simulink model "simulation code"  (R2023a)
settings: Solver=VariableStepAuto  StartTime=0.0  StopTime=1  MaxStep=1e-6  RelTol=1e-3
InitFcn:
  | Ts=1/1550;
undefined symbols (not defined in the file): powergui, sps_lib
libraries: spsIGBTDiodeLib x6, spsVoltageMeasurementLib x6, spsabctoAlphaBetaZeroLib x2, spsDCVoltageSourceLib x1, spsGroundLib x1, simulink x1, simulink_extras x1, spspowerguiLib x1, spsThreePhaseSeriesRLCBranchLib x1, spsThreePhaseVIMeasurementLib x1
settings DataIOCC: ReturnWorkspaceOutputs=off

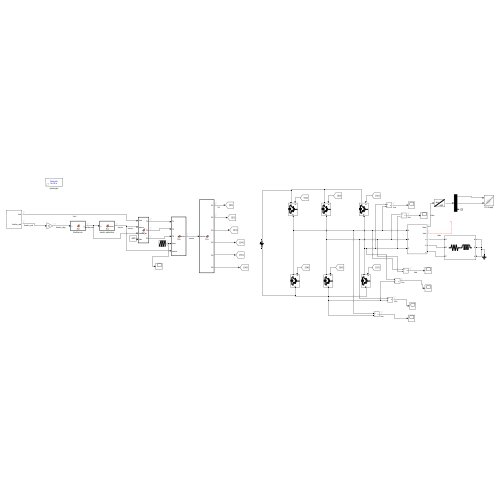
[thumbnail: Simulink's stored preview of the top-level diagram]
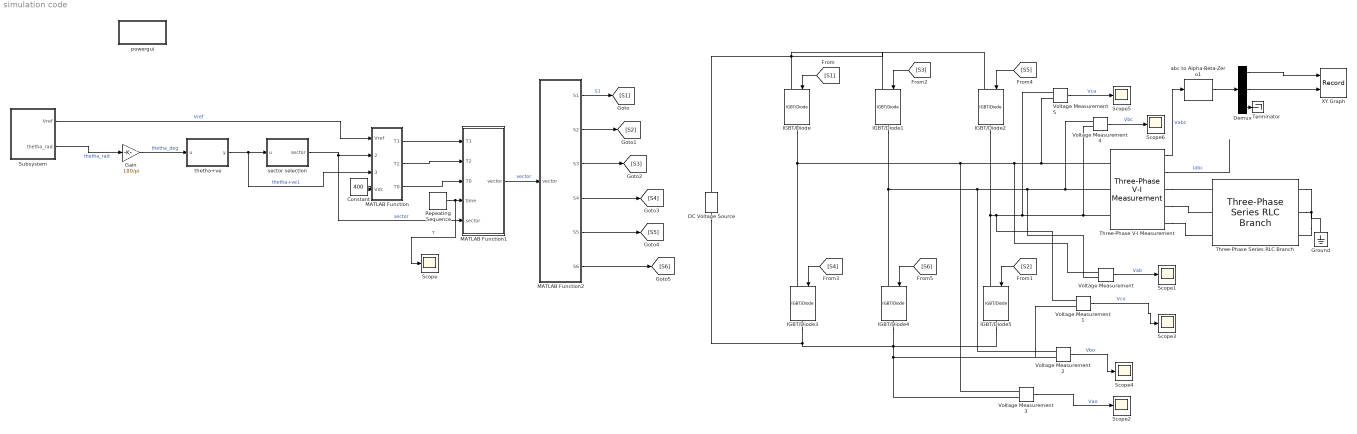
== system simulation code ==
  Constant : Constant  Value=400
  DC Voltage Source : spsDCVoltageSourceLib/DC Voltage Source  Amplitude=400  Measurements=None
  Demux : Demux  Outputs=3
  Gain : Gain  Gain=180/pi
  Ground : spsGroundLib/Ground  LConnTagsString=a
  IGBT/Diode{,1..5} (6 alike) : spsIGBTDiodeLib/IGBT//Diode  Ron=1e-3  Rs=1e5  Cs=inf  Measurements=off
  MATLAB Function : MATLAB Function  TreatAsAtomicUnit=on
  MATLAB Function1 : MATLAB Function  TreatAsAtomicUnit=on
  MATLAB Function2 : MATLAB Function  TreatAsAtomicUnit=on
  Repeating Sequence : simulink/Sources/Repeating Sequence  rep_seq_t=[0 1]*Ts  rep_seq_y=[0 Ts]
  Scope{,1..6} (7 alike) : Scope
  Subsystem : Subsystem
  Terminator : Terminator
  Three-Phase Series RLC Branch : spsThreePhaseSeriesRLCBranchLib/Three-Phase Series RLC Branch  LConnTagsString=A|B|C  RConnTagsString=A|B|C  BranchType=RL  Resistance=1  Inductance=1e-2  Capacitance=0  Measurements=None
  Three-Phase V-I Measurement : spsThreePhaseVIMeasurementLib/Three-Phase V-I Measurement  VoltageMeasurement=phase-to-ground  SetLabelV=off  LabelV=Vabc  Vpu=off  VpuLL=off  CurrentMeasurement=yes  SetLabelI=off  LabelI=Iabc  Ipu=off  Pbase=100e6  Vbase=500e3  OutputType=Complex  PhasorSimulation=off  PSBequivalent=0
  Voltage Measurement{,1..5} (6 alike) : spsVoltageMeasurementLib/Voltage Measurement  PhasorSimulation=off  OutputType=Complex  PSBequivalent=0
  XY Graph : Record  FileSettingsInternal="{\"entries\":[{\"content\":{\"excelSettings\":{\"content\":{},\"type\":\"Streamout.ExcelSettings\"}},\"type\":\"Streamout.FileSettingStorage\",\"uuid\":\"\"}],\"packageUris\":[\"http:\\/\\/schema.mathworks.com\\/mf0\\/streamout_blocks\\/R2020a\"],\"version\":\"1.0\"}"  Layout=[1 1]  SignalsInternal="{\"entries\":[{\"content\":{\"signals\":[{\"content\":{\"blockPath\":[],\"dimensions\":[1],\"domain\":\"\",\"lineColor\":\"#77ac30\",\"plots\":[1],\"port\":1,\"signalID\":12102,\"signalName\":\"Demux:1\"},\"type\":\"RecordBlkView.Signal\",\"uuid\":\"\"},{\"content\":{\"blockPath\":[],\"dimensions\":[1],\"domain\":\"\",\"lineColor\":\"#139fff\",\"plots\":[1],\"port\":2,\"signalID\":12105,\"signalName\":\"Demux:2\"},\"type\":\"RecordBlkView.Signal\",\"uuid\":\"\"}]},\"type\":\"RecordBlkView.InputSignals\",\"uuid\":\"\"}],\"packageUris\":[\"http:\\/\\/schema.mathworks.com\\/mf0\\/streamout_blocks\\/R2020a\"],\"version\":\"1.0\"}"  VisualizationBindings="{\"xyplotplugin\":{\"info\":[{\"series\":[{\"bindingParametersList\":[{\"parameter\":\"X-Axis\",\"signalID\":12102,\"signalName\":\"Demux:1\"},{\"parameter\":\"Y-Axis\",\"signalID\":12105,\"signalName\":\"Demux:2\"}],\"seriesID\":46144}],\"subplotID\":1}]}}"  CompatibilityTag=XY  st=-1
  abc to Alpha-Beta-Zero1 : spsabctoAlphaBetaZeroLib/abc to Alpha-Beta-Zero
  powergui : Subsystem  Priority=1  AncestorBlock=sps_lib/powergui  DialogController=POWERSYS.PowerSysDialog  InitFcn=powergui( 'InitFcn_Callback' , gcb , 0 , [ ] );  mask(PSB option menu block){SimulationMode=Discrete, SampleTime=50e-6, frequency=60, Iterations=50, frequencyindice=0, Pbase=100e6, ErrMax=1e-4, UnitsV=kV, UnitsW=MW, buscounter=0, FunctionMessages=off, echomessages=off, EnableUseOfTLC=off, CurrentSourceSwitches=off, DisableSnubberDevices=off, DisableRonSwitches=off, DisableVfSwitches=off, DisplayEquations=off, AutomaticDiscreteSolvers=off, SolverType=Tustin/Backward Euler (TBE), Interpol=off, ExternalGateDelay=off, methode=off, Ts=100, x0status=blocks, SPID=on, SwTol=0, HookPort=off, NonlinearTolerance=1e-4, nMaxIteration=100, ContinueOnMaxIteration=off, RestoreLinks=warning, ResistiveCurrentMeasurement=off, Frange=[0:2:500], Ylog=off, Xlog=on, ShowGrid=off, save=off, variable=ZData, structure=0, ZoomFFT=off, StartTime=0.0, cycles=1, DisplayStyle=1, fundamental=60, FreqAxis=off, MaxFrequency=1000, frequencyindicesteady=1, RmsSteady=1, display=off}
      mask prompts: SimulationMode "Simulation type:"; SampleTime "Sample time (s):"; frequency "Frequency (Hz):"; Iterations "Max iterations"; frequencyindice "Frequency (Hz)"; Pbase "Base power (VA)"; ErrMax "PQ tolerance (pu)"; UnitsV "Voltage units"; UnitsW "Power units"; buscounter "Load flow bus counter"; FunctionMessages "Disable Specialized Power Systems warnings"; echomessages "Display Specialized Power Systems compilation messages"; EnableUseOfTLC "Use TLC file when in Accelerator Simulation Mode and for code generation"; CurrentSourceSwitches "Disable ideal switching"; DisableSnubberDevices "Disable snubbers in switching devices"; DisableRonSwitches "Disable Ron resistances in switching devices"; DisableVfSwitches "Disable forward voltages in switching devices"; DisplayEquations "Display circuit differential equations"; AutomaticDiscreteSolvers "Automatically handle Discrete solver and Advanced tab solver settings of blocks"; SolverType "Discrete solver"; Interpol "Interpolate switching events"; ExternalGateDelay "Use time-stamped gate signals"; methode "Store switching topologies"; Ts "Buffer size (MBytes):"; x0status "Start simulation with initial electrical states from:"; SPID "Use ideal switching devices"; SwTol "Switch tolerance"; HookPort "Allow multiple powergui blocks"; NonlinearTolerance "Solver tolerance"; nMaxIteration "Maximum number of iterations"; ContinueOnMaxIteration "Continue Simulation if maximum number of iterations is reached"; RestoreLinks "Restore disabled links of Simscape Power Systems ST blocks:"; ResistiveCurrentMeasurement "Use non ideal current measurement blocks (1e-4Ohm internal resistance)"; Frange "Frequency Range"; Ylog "Log impedance"; Xlog "log Frequency"; ShowGrid "grid"; save "Save Data To Workspace"; variable "Variable Name"; structure "Structure Name (PSBFFTSCOPE)"; ZoomFFT "ZoomFFT (PSBFFTSCOPE)"; StartTime "Start Time (PSBFFTSCOPE)"; cycles "Cycles (PSBFFTSCOPE)"; DisplayStyle "Display style (PSBFFTSCOPE)"; fundamental "Fundamental (PSBFFTSCOPE)"; FreqAxis "Frequency Axis (PSBFFTSCOPE)"; MaxFrequency "Max Frequency (PSBFFTSCOPE)"; frequencyindicesteady "Frequency indice (STEADYSTATE)"; RmsSteady "RMS display (STEADYSTATE)"; display "Display Results"
      mask help: Set simulation type, simulation parameters, and preferences.
      mask init:
      | dispMessage = '';
      | dispMessage = powergui('MaskInitialization',gcb,SimulationMode,SampleTime);
      settings: LibrarySourceBlock=sps_lib/powergui  PreSaveFcn=powergui( 'PreSaveFcn_Callback' , gcb , [ ] , [ ] );  OpenFcn=sps_rtmsupport('OpenFcn',gcbh)
      mask Help: helpview(psbhelp)
      mask TypeOptions SimulationMode: Continuous | Discrete | Phasor | Discrete phasor
      mask Callback SimulationMode: powergui('SimulationType',[],[],gcb);
      mask TypeOptions UnitsV: V | kV
      mask TypeOptions UnitsW: W | kW | MW
      mask Callback CurrentSourceSwitches: powergui('SimulationType',[],[],gcb);
      mask Callback AutomaticDiscreteSolvers: powergui('SimulationType',[],[],gcb);
      mask TypeOptions SolverType: Tustin/Backward Euler (TBE) | Tustin | Backward Euler
      mask Callback SolverType: powergui('SimulationType',[],[],gcb);
      mask Callback Interpol: powergui('SimulationType',[],[],gcb);
      mask Callback ExternalGateDelay: powergui('SimulationType',[],[],gcb);
      mask Callback methode: powergui('SimulationType',[],[],gcb);
      mask TypeOptions x0status: blocks | steady | zero
      mask TypeOptions RestoreLinks: yes | warning | no
      mask Callback display: sps_rtmsupport('parametereditingmodes',gcbh) % Will be executed last in parameter callbacks to ensure mask enable consistency
      mask DialogControl SolverTab Prompt: Solver
      mask DialogControl AutoSolverNote Prompt: The Simulation type parameter is governed by Simulink. To access the Powergui solver settings, unselect auto (Automatic solver selection) solver in the Simulink solver options.
      mask DialogControl Apps Prompt: Apps
      mask DialogControl StateAnalyzer Prompt: Measurements and States Analyzer
      mask DialogControl StateAnalyzer Callback: powerStates(bdroot(gcb))
      mask DialogControl LineParameterCalculator Prompt: Line Parameter Calculator
      mask DialogControl LineParameterCalculator Callback:
      | close_system(gcb)
      | powerLineParameters
      mask DialogControl CableParameterCalculator Prompt: Cable Parameter Calculator
      mask DialogControl CableParameterCalculator Callback:
      | close_system(gcb)
      | powerCableParameters
      mask DialogControl LineDecoupler Prompt: Line Decoupler
      mask DialogControl LineDecoupler Tooltip: Click to replace selected Distributed Parameters Line blocks with Decoupling Line blocks
      mask DialogControl LineDecoupler Callback:
      | close_system(gcb);
      | DecouplingLineReplace(gcs)
      mask DialogControl LoadFlowAnalyzer Prompt: Load Flow Analyzer
      mask DialogControl LoadFlowAnalyzer Callback:
      | close_system(gcb)
      | powerLoadFlow
      mask DialogControl LoadFlowParameters Prompt: Load Flow Parameters
      mask DialogControl ImpedanceCalculator Prompt: Impedance Calculator
      mask DialogControl ImpedanceCalculator Callback:
      | close_system(gcb);
      | powerImpedance(bdroot(gcs));
      mask DialogControl FFTAnalyzer Prompt: FFT Analyzer
      mask DialogControl FFTAnalyzer Callback:
      | close_system(gcb)
      | power_fftscope(bdroot(gcb),gcb)
      mask DialogControl LinearSystemAnalyzer Prompt: Linear System Analyzer
      mask DialogControl LinearSystemAnalyzer Callback:
      | close_system(gcb)
      | power_ltiview(bdroot(gcb))
      mask DialogControl HysteresisDesigner Prompt: Hysteresis Designer
      mask DialogControl HysteresisDesigner Callback:
      | close_system(gcb)
      | powerHysteresis('hysteresis.mat')
      mask DialogControl BlockCustomizer Prompt: Block Customizer
      mask DialogControl BlockCustomizer Callback:
      | close_system(gcb);
      | power_customize;
      mask DialogControl ReportGenerator Prompt: Report Generator
      mask DialogControl ReportGenerator Callback:
      | close_system(gcb)
      | power_report(bdroot(gcb))
      mask DialogControl obsolete Prompt: ...
      mask DialogControl MachineInitialization Prompt: Machine Initialization
      mask DialogControl MachineInitialization Callback:
      | close_system(gcb)
      | powericon('machineInitTool',bdroot(gcb),gcb)
      mask DialogControl Preferences Prompt: Preferences
      mask DialogControl Solver Prompt: Solver
      mask DialogControl SolverDetails Prompt: Solver details for nonlinear elements
      mask Display: color('blue'),disp(dispMessage)
  sector selection : MATLAB Function  TreatAsAtomicUnit=on
  thetha+ve : MATLAB Function  TreatAsAtomicUnit=on
  wires:
  Subsystem/2(thetha_rad) -> Gain/1  "thetha_rad"
  Gain/1 -> thetha+ve/1(u)  "thetha_deg"
  thetha+ve/1(y) -> MATLAB Function/3(thetha_ve), sector selection/1(u)  "thetha+ve1"
  sector selection/1(sector) -> MATLAB Function1/5(sector), MATLAB Function/2(sector)  "sector"
  Subsystem/1(Vref) -> MATLAB Function/1(Vref)  "Vref"
  Constant/1 -> MATLAB Function/4(Vdc)
  MATLAB Function/1(T1) -> MATLAB Function1/1(T1)
  MATLAB Function/2(T2) -> MATLAB Function1/2(T2)
  MATLAB Function/3(T0) -> MATLAB Function1/3(T0)
  Repeating Sequence/1 -> Scope/1, MATLAB Function1/4(time)  "T"
  MATLAB Function1/1(vector) -> MATLAB Function2/1(vector)  "vector"
  MATLAB Function2/1(S1) -> [S1]  "S1"
  MATLAB Function2/2(S2) -> [S2]
  MATLAB Function2/3(S3) -> [S3]
  MATLAB Function2/6(S6) -> [S6]
  MATLAB Function2/4(S4) -> [S4]
  MATLAB Function2/5(S5) -> [S5]
  [S1] -> IGBT/Diode/1
  [S3] -> IGBT/Diode1/1
  [S5] -> IGBT/Diode2/1
  [S2] -> IGBT/Diode5/1
  [S6] -> IGBT/Diode4/1
  [S4] -> IGBT/Diode3/1
  Three-Phase V-I Measurement/1 -> abc to Alpha-Beta-Zero1/1  "Vabc"
  abc to Alpha-Beta-Zero1/1 -> Demux/1
  Demux/1 -> XY Graph/1
  Demux/2 -> XY Graph/2
  Demux/3 -> Terminator/1
  Voltage Measurement/1 -> Scope1/1  "Vab"
  Voltage Measurement1/1 -> Scope3/1  "Vco"
  Voltage Measurement2/1 -> Scope4/1  "Vbo"
  Voltage Measurement3/1 -> Scope2/1  "Vao"
  Three-Phase V-I Measurement/2 -> ?  "Iabc"
  Voltage Measurement5/1 -> Scope5/1  "Vca"
  Voltage Measurement4/1 -> Scope6/1  "Vbc"
  connections:
  Three-Phase V-I Measurement/LConn1 -- Voltage Measurement5/LConn2 -- Voltage Measurement/LConn1 -- IGBT/Diode3/LConn1 -- IGBT/Diode/RConn1 -- Voltage Measurement3/LConn1
  Three-Phase V-I Measurement/LConn2 -- Voltage Measurement4/LConn1 -- Voltage Measurement/LConn2 -- Voltage Measurement2/LConn1 -- IGBT/Diode4/LConn1 -- IGBT/Diode1/RConn1
  Three-Phase V-I Measurement/LConn3 -- Voltage Measurement4/LConn2 -- Voltage Measurement5/LConn1 -- Voltage Measurement1/LConn1 -- IGBT/Diode5/LConn1 -- IGBT/Diode2/RConn1
  IGBT/Diode2/LConn1 -- IGBT/Diode1/LConn1 -- IGBT/Diode/LConn1 -- DC Voltage Source/RConn1
  DC Voltage Source/LConn1 -- IGBT/Diode3/RConn1 -- Voltage Measurement1/LConn2 -- Voltage Measurement2/LConn2 -- Voltage Measurement3/LConn2 -- IGBT/Diode5/RConn1 -- IGBT/Diode4/RConn1
  Three-Phase Series RLC Branch/RConn1 -- Three-Phase Series RLC Branch/RConn3 -- Ground/LConn1 -- Three-Phase Series RLC Branch/RConn2
  Three-Phase V-I Measurement/RConn1 -- Three-Phase Series RLC Branch/LConn1
  Three-Phase V-I Measurement/RConn2 -- Three-Phase Series RLC Branch/LConn2
  Three-Phase V-I Measurement/RConn3 -- Three-Phase Series RLC Branch/LConn3

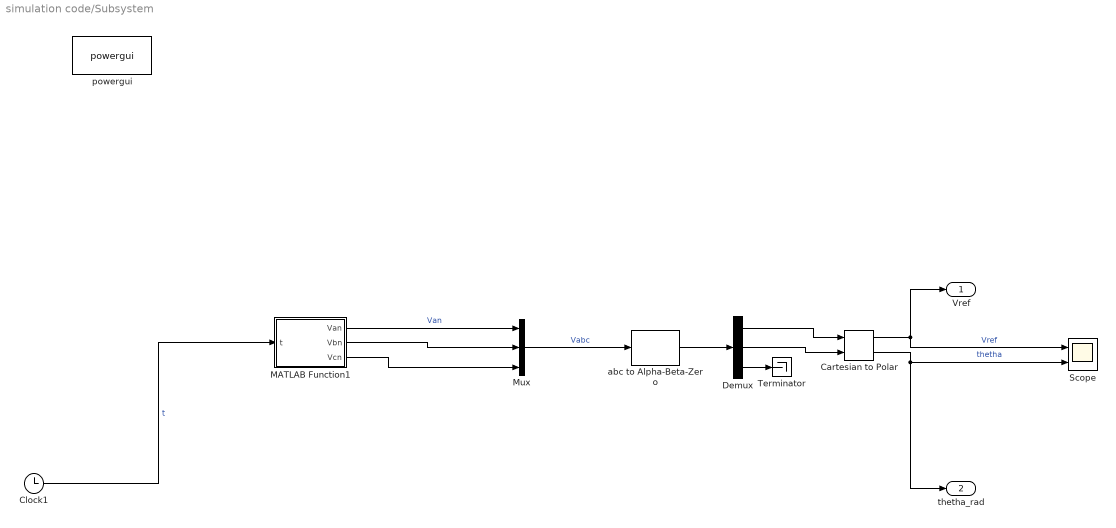
== system simulation code/Subsystem ==
  Cartesian to Polar : simulink_extras/Transformations/Cartesian to Polar
  Clock1 : Clock
  Demux : Demux  Outputs=3
  MATLAB Function1 : MATLAB Function  TreatAsAtomicUnit=on
  Mux : Mux  Inputs=3
  Scope : Scope  NumInputPorts=2
  Terminator : Terminator
  abc to Alpha-Beta-Zero : spsabctoAlphaBetaZeroLib/abc to Alpha-Beta-Zero
  powergui : spspowerguiLib/powergui  Priority=1  SimulationMode=Discrete  SampleTime=50e-6  frequency=60  Iterations=50  frequencyindice=60  Pbase=100e6  ErrMax=1e-4  UnitsV=kV  UnitsW=MW  buscounter=0  FunctionMessages=off  echomessages=off  EnableUseOfTLC=off  CurrentSourceSwitches=off  DisableSnubberDevices=off  DisableRonSwitches=off  DisableVfSwitches=off  DisplayEquations=off  AutomaticDiscreteSolvers=off  SolverType=Tustin/Backward Euler (TBE)  Interpol=off  ExternalGateDelay=off  methode=off  Ts=100  x0status=blocks  SPID=on  SwTol=0  HookPort=off  NonlinearTolerance=1e-4  nMaxIteration=100  ContinueOnMaxIteration=off  RestoreLinks=warning  ResistiveCurrentMeasurement=off  Frange=[0:2:500]  Ylog=off  Xlog=on  ShowGrid=off  save=off  variable=ZData  structure=0  ZoomFFT=off  StartTime=0.0  cycles=1  DisplayStyle=1  fundamental=60  FreqAxis=off  MaxFrequency=1000  frequencyindicesteady=1  RmsSteady=1  display=off
  Vref : Outport
  thetha_rad : Outport  Port=2
  wires:
  Mux/1 -> abc to Alpha-Beta-Zero/1  "Vabc"
  abc to Alpha-Beta-Zero/1 -> Demux/1
  Demux/1 -> Cartesian to Polar/1
  Demux/2 -> Cartesian to Polar/2
  Cartesian to Polar/1 -> Vref/1, Scope/1  "Vref"
  Cartesian to Polar/2 -> thetha_rad/1, Scope/2  "thetha"
  Clock1/1 -> MATLAB Function1/1(t)  "t"
  MATLAB Function1/3(Vcn) -> Mux/3
  MATLAB Function1/2(Vbn) -> Mux/2
  MATLAB Function1/1(Van) -> Mux/1  "Van"
  Demux/3 -> Terminator/1

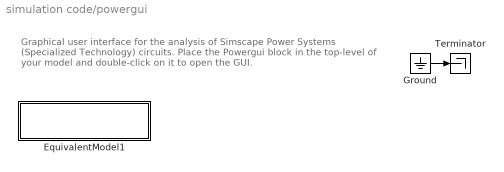
== system simulation code/powergui ==
  note: Graphical user interface for the analysis of
      | Simscape Power Systems (Specialized Technology) circuits.
      | Place the Powergui block in the top-level of your model and double-click
      | on it to open the GUI.
  EquivalentModel1 : Subsystem
      mask init:
      | S  = GetDataForEquivalentModel('Discrete',gcbh);
      mask Display:
      | color('red')
      | disp('EQUIVALENT CIRCUIT\nDiscrete')
  Ground : Ground
  Terminator : Terminator
  wires:
  Ground/1 -> Terminator/1

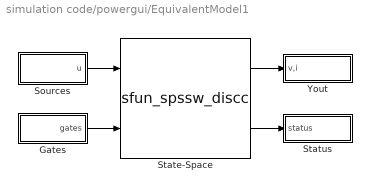
== system simulation code/powergui/EquivalentModel1 ==
  Gates : Subsystem
  Sources : Subsystem
  State-Space : S-Function  FunctionName=sfun_spssw_discc  Parameters=S.Ts,S.A, S.B, S.C, S.D, S.x0, S.EnableUseOfTLC,S.SwitchResistance ,S.SwitchType, S.SwitchGateInitialValue, S.OutputsToResetToZero, S.TBEON,S.SaveMatrices,S.BufferSize  SFunctionDeploymentMode=off  EnableBusSupport=off
  Status : Subsystem
  Yout : Subsystem
  wires:
  Gates/1(gates) -> State-Space/2
  Sources/1(u) -> State-Space/1
  State-Space/2 -> Status/1(status)
  State-Space/1 -> Yout/1(v,i)

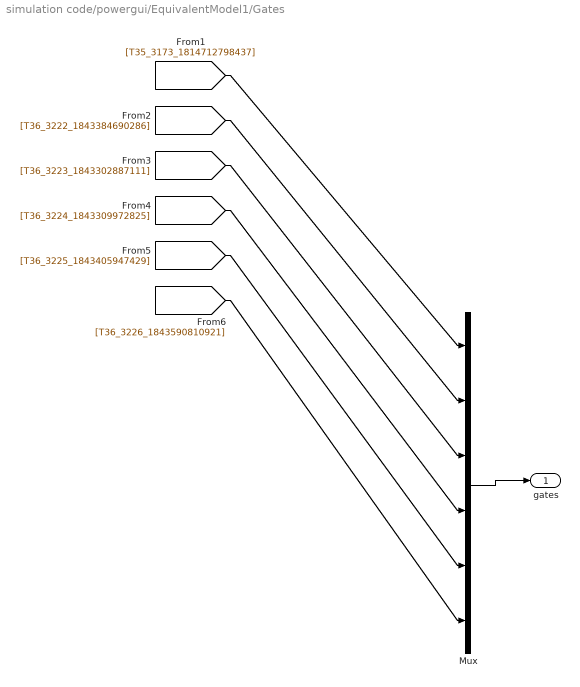
== system simulation code/powergui/EquivalentModel1/Gates ==
  Mux : Mux  Inputs=[1 1 1 1 1 1]
  gates : Outport  VectorParamsAs1DForOutWhenUnconnected=off
  wires:
  Mux/1 -> gates/1
  [T35_3173_1814712798437] -> Mux/1
  [T36_3222_1843384690286] -> Mux/2
  [T36_3223_1843302887111] -> Mux/3
  [T36_3224_1843309972825] -> Mux/4
  [T36_3225_1843405947429] -> Mux/5
  [T36_3226_1843590810921] -> Mux/6

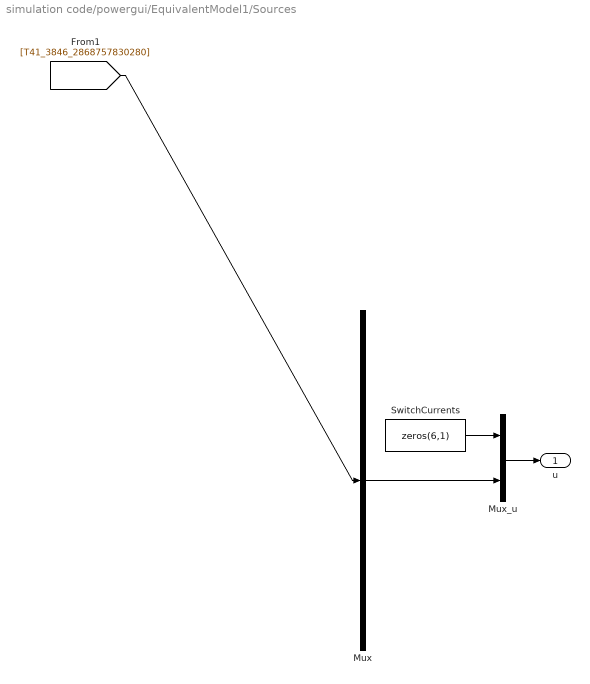
== system simulation code/powergui/EquivalentModel1/Sources ==
  Mux : Mux  Inputs=1
  Mux_u : Mux  Inputs=[6 1]
  SwitchCurrents : Constant  Value=zeros(6,1)
  u : Outport  VectorParamsAs1DForOutWhenUnconnected=off
  wires:
  Mux_u/1 -> u/1
  SwitchCurrents/1 -> Mux_u/1
  Mux/1 -> Mux_u/2
  [T41_3846_2868757830280] -> Mux/1

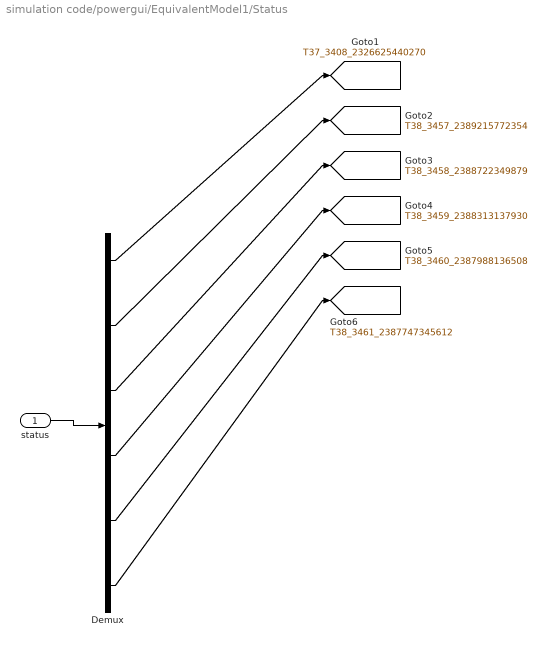
== system simulation code/powergui/EquivalentModel1/Status ==
  status : Inport
  Demux : Demux  Outputs=[1 1 1 1 1 1]
  tag scope: T37_3408_2326625440270=global, T38_3457_2389215772354=global, T38_3458_2388722349879=global, T38_3459_2388313137930=global, T38_3460_2387988136508=global, T38_3461_2387747345612=global
  wires:
  status/1 -> Demux/1
  Demux/1 -> [T37_3408_2326625440270]
  Demux/2 -> [T38_3457_2389215772354]
  Demux/3 -> [T38_3458_2388722349879]
  Demux/4 -> [T38_3459_2388313137930]
  Demux/5 -> [T38_3460_2387988136508]
  Demux/6 -> [T38_3461_2387747345612]

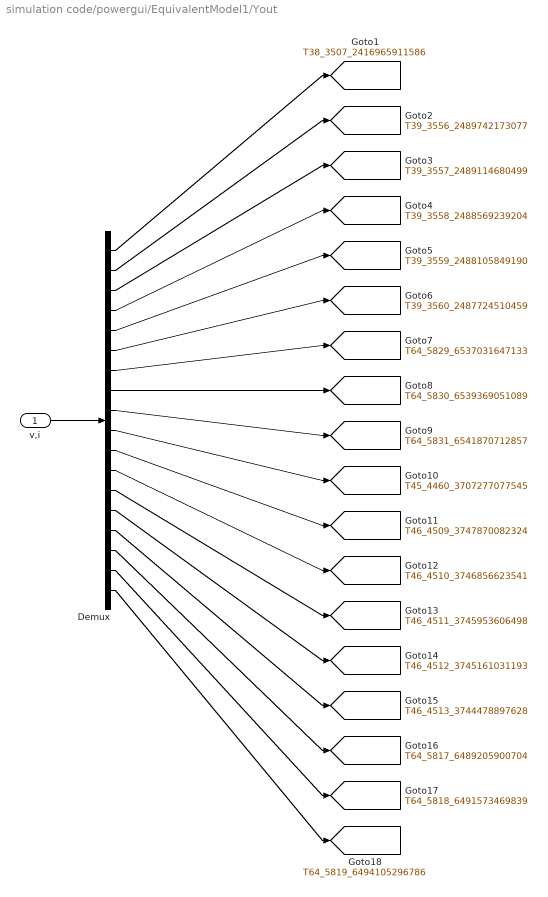
== system simulation code/powergui/EquivalentModel1/Yout ==
  v,i : Inport
  Demux : Demux  Outputs=[1 1 1 1 1 1 1 1 1 1 1 1 1 1 1 1 1 1]
  tag scope: T38_3507_2416965911586=global, T39_3556_2489742173077=global, T39_3557_2489114680499=global, T39_3558_2488569239204=global, T39_3559_2488105849190=global, T39_3560_2487724510459=global, T45_4460_3707277077545=global, T46_4509_3747870082324=global, T46_4510_3746856623541=global, T46_4511_3745953606498=global, T46_4512_3745161031193=global, T46_4513_3744478897628=global, T64_5817_6489205900704=global, T64_5818_6491573469839=global, T64_5819_6494105296786=global, T64_5829_6537031647133=global, T64_5830_6539369051089=global, T64_5831_6541870712857=global
  wires:
  v,i/1 -> Demux/1
  Demux/1 -> [T38_3507_2416965911586]
  Demux/2 -> [T39_3556_2489742173077]
  Demux/3 -> [T39_3557_2489114680499]
  Demux/4 -> [T39_3558_2488569239204]
  Demux/5 -> [T39_3559_2488105849190]
  Demux/6 -> [T39_3560_2487724510459]
  Demux/7 -> [T64_5829_6537031647133]
  Demux/8 -> [T64_5830_6539369051089]
  Demux/9 -> [T64_5831_6541870712857]
  Demux/10 -> [T45_4460_3707277077545]
  Demux/11 -> [T46_4509_3747870082324]
  Demux/12 -> [T46_4510_3746856623541]
  Demux/13 -> [T46_4511_3745953606498]
  Demux/14 -> [T46_4512_3745161031193]
  Demux/15 -> [T46_4513_3744478897628]
  Demux/16 -> [T64_5817_6489205900704]
  Demux/17 -> [T64_5818_6491573469839]
  Demux/18 -> [T64_5819_6494105296786]

== matlab function simulation code/thetha+ve ==
  data: u input; y output
function y = fcn(u)
angle=u(1);
if (angle>=0)
    y=angle;
else
    y=angle+360;
end

== matlab function simulation code/sector selection ==
  data: u input; sector output
function sector= fcn(u)
angle=u(1);
if (angle>=0)&&(angle<60)
    sector=1;
elseif (angle>=60)&&(angle<120)
    sector=2;
elseif (angle>=120)&&(angle<180)
    sector=3;
elseif (angle>=180)&&(angle<240)
    sector=4;
elseif (angle>=240)&&(angle<300)
    sector=5;
else
    sector=6;
end

== matlab function simulation code/MATLAB Function ==
  data: Vref input; sector input; T1 output; thetha_ve input; Vdc input; T2 output; T0 output
function [T1,T2,T0] = fcn(Vref,sector,thetha_ve,Vdc)
Ma=sqrt(3)*Vref/Vdc;
thetha=thetha_ve*pi/180;
K=sector;
Ts=1/1550;
THETHA1=thetha-(K-1)*pi/3;
T1=Ma*Ts*sin((pi/3)-THETHA1);
T2=Ma*Ts*sin(THETHA1);
T0=Ts-T1-T2;
end

== matlab function simulation code/MATLAB Function1 ==
  data: T1 input; vector output; T2 input; T0 input; time input; sector input
function vector  = fcn(T1,T2,T0,time,sector)
tt1=T0/4;
tt2=tt1+T2/2;
tt3=tt2+T1/2;
tt4=tt3+T0/2;
tt5=tt4+T1/2;
tt6=tt5+T2/2;

t1=T0/4;
t2=t1+T1/2;
t3=t2+T2/2;
t4=t3+T0/2;
t5=t4+T2/2;
t6=t5+T1/2;
if sector==1
    if (time<=tt1)&&(time>0)
        vector=7;
    elseif(time<=tt2)&&(time>tt1)
        vector=2;
    elseif (time<=tt3)&&(time>tt2)
        vector=1;
    elseif (time<=tt4)&&(time>tt3)
        vector=8;
    elseif (time<=tt5)&&(time>tt4)
        vector=1;
    elseif (time<=tt6)&&(time>tt5)
        vector=2;
    else
        vector=7;
    end
elseif sector==2
    if(time<=t1)&&(time>0)
        vector=7;
    elseif (time<=t2)&&(time>t1)
        vector=2;
    elseif (time<=t3)&&(time>t2)
        vector=3;
    elseif(time<=t4)&&(time>t3)
        vector=8;
    elseif (time<=t5)&&(time>t4)
        vector=3;
    elseif(time<=t6)&&(time>t5)
        vector=2;
    else
        vector=7;
    end
elseif sector==3
    if(time<=tt1)&&(time>0)
vector=7;
    elseif(time<=tt2)&&(time>tt1)
        vector=4;
    elseif (time<=tt3)&&(time>tt2)
        vector=3;
    elseif (time<=tt4)&&(time>=tt3)
        vector=8;
    elseif(time<=tt5)&&(time>tt4)
        vector=3;
    elseif (time<=tt6)&&(time>tt5)
        vector=4;
    else
        vector=7;
    end
elseif sector==4
    if (time<=t1)&&(time>0)
        vector=7;
    elseif (time<=t2)&&(time>t1)
        vector=4;
    elseif (time<=t3)&&(time>t2)
        vector=5;
    elseif (time<=t4)&&(time>t3)
        vector=8;
    elseif (time<=t5)&&(time>t4)
        vector=5;
    elseif(time<=t6)&&(time>t5)
        vector=4;
    else
        vector=7;
    end
elseif sector==5
    if(time<=tt1)&&(time>0)
        vector=7;
    elseif (time<=tt2)&&(time>tt1)
        vector=6;
    elseif (time<=tt3)&&(time>tt2)
        vector=5;
    elseif(time<=tt4)&&(time>tt3)
        vector=8;
    elseif(time<=tt5)&&(time>tt4)
        vector=5;
    elseif(time<=tt6)&&(time>tt5)
        vector=6;
    else
        vector=7;
    end
else
    if(time<=t1)&&(time>0)
        vector=7;
    elseif (time<=t2)&&(time>t1)
        vector=6;
    elseif(time<=t3)&&(time>t2)
        vector=1;
    elseif (time<=t4)&&(time>t3)
        vector=8;
    elseif (time<=t5)&&(time>t4)
        vector=1;
    elseif(time<=t6)&&(time>t5)
        vector=6;
    else
        vector=7;
    end
end
end

== matlab function simulation code/MATLAB Function2 ==
  data: vector input; S1 output; S2 output; S3 output; S4 output; S5 output; S6 output
function [S1,S2,S3,S4, S5,S6]= fcn(vector)
if vector==8
    S1=0;
    S2=1;
   S3=0;
   S4=1;
   S5=0;
   S6=1;
elseif vector==7
    S1=1;
    S2=0;
    S3=1;
    S4=0;
    S5=1;
    S6=0;
elseif vector==6
    S1=1;
    S2=0;
    S3=0;
    S4=0;
    S5=1;
    S6=1;
elseif vector==5
    S1=0;
    S2=0;
    S3=0;
    S4=1;
    S5=1;
    S6=1;
elseif vector==4
    S1=0;
    S2=0;
    S3=1;
    S4=1;
    S5=1;
    S6=0;
elseif vector==3
    S1=0;
    S2=1;
    S3=1;
    S4=1;
    S5=0;
    S6=0;
elseif vector==2
    S1=1;
    S2=1;
    S3=1;
    S4=0;
    S5=0;
    S6=0;
else
    S1=1;
    S2=1;
    S3=0;
    S4=0;
    S5=0;
    S6=1;
end
end

== matlab function simulation code/Subsystem/MATLAB Function1 ==
  data: t input; Van output; Vbn output; Vcn output
function [Van,Vbn,Vcn]= fcn(t)


w=2*pi*50;
thetha1=2*pi/3;
thetha2=4*pi/3;
Van=400/sqrt(3)*sin(w*t);
Vbn=400/sqrt(3)*sin(w*t-thetha1);
Vcn=400/sqrt(3)*sin(w*t-thetha2);
end
